simulink model "accel_command_smoothing_saturation"  (R2024a)
settings: Solver=FixedStepDiscrete  StartTime=0.0  StopTime=10.0  FixedStep=0.05  RelTol=1e-3
undefined symbols (not defined in the file): simStepSize
settings Model: Creator=darkh  LastModifiedBy=darkh
settings OptimizationCC: ZeroExternalMemoryAtStartup=off  ZeroInternalMemoryAtStartup=off
settings RTWCC: Description=Generate an RTMaps component embedding the model  SystemTargetFile=rtmaps.tlc  TemplateMakefile=rtmaps_default_tmf  PostCodeGenCommand=rtmaps_post_code_generation(buildInfo)  RetainRTWFile=on  TargetLang=C++
settings STFCustomTargetCC: TargetLangStandard=C++11 (ISO)  ModelReferenceCompliant=off  ConcurrentExecutionCompliant=on  CombineOutputUpdateFcns=on  CodeInterfacePackaging=C++ class  CPPClassGenCompliant=on  GRTInterface=off  UseToolchainInfoCompliant=off  SystemTargetFile=rtmaps.tlc
settings GRTTargetCC: TargetLangStandard=C++11 (ISO)  ModelReferenceCompliant=off  ParMdlRefBuildCompliant=off  CompOptLevelCompliant=off  MatFileLogging=off  CodeInterfacePackaging=C++ class  UseToolchainInfoCompliant=off

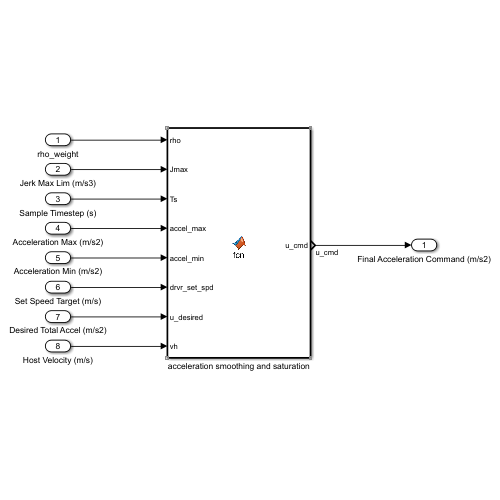
[thumbnail: Simulink's stored preview of the top-level diagram]
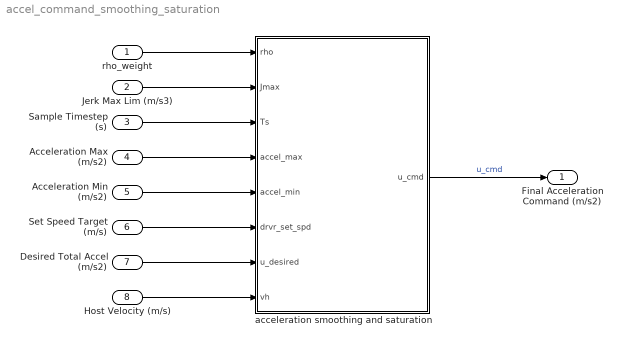
== system accel_command_smoothing_saturation ==
  rho_weight : Inport
  Jerk Max Lim (m/s3) : Inport  Port=2
  Sample Timestep (s) : Inport  Port=3
  Acceleration Max (m/s2) : Inport  Port=4
  Acceleration Min (m/s2) : Inport  Port=5
  Set Speed Target (m/s) : Inport  Port=6
  Desired Total Accel (m/s2) : Inport  Port=7
  Host Velocity (m/s) : Inport  Port=8
  acceleration smoothing and saturation : MATLAB Function  TreatAsAtomicUnit=on  SystemSampleTime=simStepSize
  Final Acceleration Command (m/s2) : Outport
  wires:
  rho_weight/1 -> acceleration smoothing and saturation/1(rho)
  Jerk Max Lim (m/s3)/1 -> acceleration smoothing and saturation/2(Jmax)
  Sample Timestep (s)/1 -> acceleration smoothing and saturation/3(Ts)
  Acceleration Max (m/s2)/1 -> acceleration smoothing and saturation/4(accel_max)
  Acceleration Min (m/s2)/1 -> acceleration smoothing and saturation/5(accel_min)
  Set Speed Target (m/s)/1 -> acceleration smoothing and saturation/6(drvr_set_spd)
  Desired Total Accel (m/s2)/1 -> acceleration smoothing and saturation/7(u_desired)
  Host Velocity (m/s)/1 -> acceleration smoothing and saturation/8(vh)
  acceleration smoothing and saturation/1(u_cmd) -> Final Acceleration Command (m/s2)/1  "u_cmd"

== matlab function accel_command_smoothing_saturation/acceleration smoothing and saturation ==
  data: rho input; Jmax input; Ts input; accel_max input; accel_min input; drvr_set_spd input; u_cmd output; u_desired input; vh input
% function [u_cmd, here, u_k_min_1] = fcn(rho, Jmax, Ts, accel_max, accel_min, drvr_set_spd, u_desired, vh)
function u_cmd = fcn(rho, Jmax, Ts, accel_max, accel_min, drvr_set_spd, u_desired, vh)
% This function is the smoothing step that determines a commanded control
% signal based on minimizing the following QP : J(u) = (u-u_lqr)^2 + rho*(u - uk_minus_1)^2
% This block also limits the acceleration output if the vehicle is at or past the driver set speed value OR if telling car to go backwards

persistent u_k_minus_1
if isempty(u_k_minus_1)
    u_k_minus_1 = 0.0;
end

% u_k_min_1 = u_k_minus_1; % for debugginggggggg

u_tilde = (u_desired + rho*u_k_minus_1)/(1 + rho); % jerk and control deviation cost minimizing control signal

u_cmd = min(max(u_tilde, u_k_minus_1 - Jmax*Ts), u_k_minus_1 + Jmax*Ts); % rate-limiting the control signal (jerk limits)
u_cmd = min(max(u_cmd, accel_min), accel_max); % Applying acceleration magnitude limits to control signal

% here = 0; % for debugging

if (vh <= 0.001 && u_cmd < 0.0) % If vehicle is at a full stop and controller requests a negative acceleration, set commanded accel to 0 m/s^2
    u_cmd = 0.0;
    u_k_minus_1 = u_cmd; % updating previous input value for use next timestep

    % here  = 1;
    return;

elseif (vh >= drvr_set_spd-0.5 && u_cmd >= 0.0) % If vehicle is approaching driver set limit and controller requests positive accel, set command to 0 m/s^2
    u_cmd = min(max(0.0, u_k_minus_1 - Jmax*Ts), u_k_minus_1 + Jmax*Ts); % Move to 0.0 m/s^2 acceleration with maximum allowable jerk
    u_k_minus_1 = u_cmd; % updating previous input value for use next timestep
    
    % here = 2;
    return;
end

u_k_minus_1 = u_cmd; % updating previous input value for use next timestep
